simulink subsystem "block_admittance_controller_quat"  (R2021b)
settings: Solver=VariableStepAuto  StartTime=0.0  StopTime=10.0  RelTol=1e-3
undefined symbols (not defined in the file): Kd, Kp, Md, q_d_cd0, w_d_cd0
settings Model: Creator=Martin  LastModifiedBy=Martin

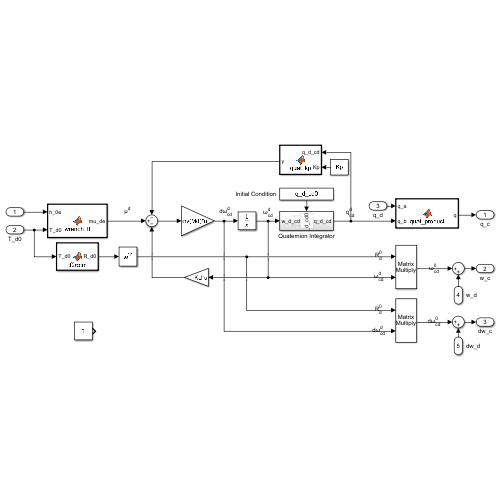
[thumbnail: Simulink's stored preview of the top-level diagram]
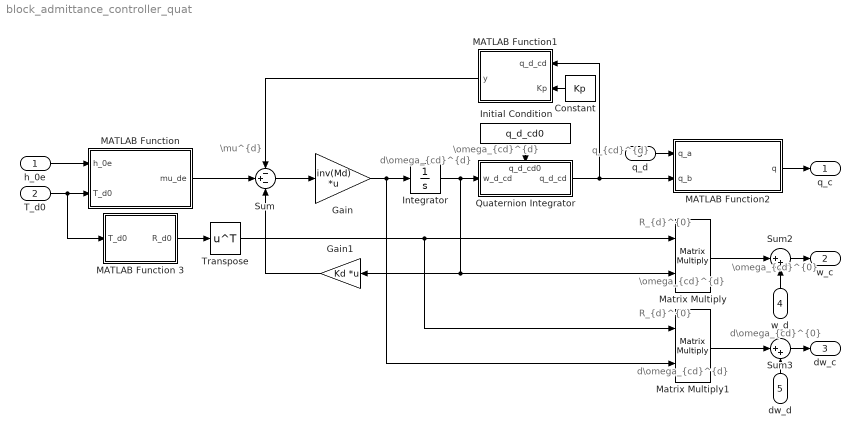
== system block_admittance_controller_quat ==
  note: q_{cd}^{d}
  note: \omega_{cd}^{d}
  note: d\omega_{cd}^{d}
  note: \omega_{cd}^{d}
  note: R_{d}^{0}
  note: \omega_{cd}^{0}
  note: \mu^{d}
  note: R_{d}^{0}
  note: d\omega_{cd}^{d}
  note: d\omega_{cd}^{0}
  h_0e : Inport
  T_d0 : Inport  Port=2
  q_d : Inport  Port=3  PortDimensions=[1 4]
  w_d : Inport  Port=4
  dw_d : Inport  Port=5
  Constant : Constant  Value=Kp  VectorParams1D=off
  Gain : Gain  Gain=inv(Md)  Multiplication=Matrix(K*u)
  Gain1 : Gain  Gain=Kd  Multiplication=Matrix(K*u)
  Initial Condition : Constant  Value=q_d_cd0  VectorParams1D=off
  Integrator : Integrator  InitialCondition=w_d_cd0
  MATLAB Function : MATLAB Function  TreatAsAtomicUnit=on
  MATLAB Function 3 : MATLAB Function  TreatAsAtomicUnit=on
  MATLAB Function1 : MATLAB Function  TreatAsAtomicUnit=on
  MATLAB Function2 : MATLAB Function  TreatAsAtomicUnit=on
  Matrix Multiply : Product  Multiplication=Matrix(*)
  Matrix Multiply1 : Product  Multiplication=Matrix(*)
  Quaternion Integrator : Subsystem
      settings: PortSchema="{\"entries\":[{\"content\":{\"sides\":[{\"content\":{\"connectorIds\":[\"In1\"]},\"type\":\"ConnectorPlacement.EquallySpacedRectSide\",\"uuid\":\"9147276c-c282-42f4-b280-5cb7655f40a2\"},{\"content\":{\"connectorIds\":[\"Out1\"],\"side\":\"RIGHT\"},\"type\":\"ConnectorPlacement.EquallySpacedRectSide\",\"uuid\":\"8158b75f-7283-43f6-a546-44f02f66480d\"},{\"content\":{\"connectorIds\":[\"In2\"],\"side\":\"TOP\"},\"type\":\"ConnectorPlacement.EquallySpacedRectSide\",\"uuid\":\"e337812f-5cf7-40c1-8c1c-b6f28ef83770\"},{\"content\":{\"connectorIds\":[],\"side\":\"BOTTOM\"},\"type\":\"ConnectorPlacement.EquallySpacedRectSide\",\"uuid\":\"6d87eade-312b-4fff-ae27-7548639e2b90\"}]},\"type\":\"ConnectorPlacement.EquallySpacedConnector\",\"uuid\":\"76e88866-094a-46fd-b80c-7282024b89fb\"}],\"packageUris\":[\"http://schema.mathworks.com/mf0/Connector/R2020b\"],\"version\":\"1.0\"}"
  Sum : Sum  Inputs=-+-
  Sum2 : Sum  Inputs=|++
  Sum3 : Sum  Inputs=|++
  Transpose : Math  Operator=transpose  SaturateOnIntegerOverflow=on
  q_c : Outport
  w_c : Outport  Port=2
  dw_c : Outport  Port=3
  wires:
  Sum2/1 -> w_c/1
  Sum3/1 -> dw_c/1
  Gain/1 -> Integrator/1, Matrix Multiply1/2
  w_d/1 -> Sum2/2
  dw_d/1 -> Sum3/2
  Sum/1 -> Gain/1
  Gain1/1 -> Sum/3
  h_0e/1 -> MATLAB Function/1(h_0e)
  MATLAB Function/1(mu_de) -> Sum/2
  T_d0/1 -> MATLAB Function/2(T_d0), MATLAB Function 3/1(T_d0)
  Quaternion Integrator/1(q_d_cd) -> MATLAB Function1/1(q_d_cd), MATLAB Function2/2(q_b)
  Initial Condition/1 -> Quaternion Integrator/2(q_d_cd0)
  MATLAB Function1/1(y) -> Sum/1
  Constant/1 -> MATLAB Function1/2(Kp)
  MATLAB Function2/1(q) -> q_c/1
  q_d/1 -> MATLAB Function2/1(q_a)
  MATLAB Function 3/1(R_d0) -> Transpose/1
  Matrix Multiply/1 -> Sum2/1
  Transpose/1 -> Matrix Multiply/1, Matrix Multiply1/1
  Integrator/1 -> Matrix Multiply/2, Gain1/1, Quaternion Integrator/1(w_d_cd)
  Matrix Multiply1/1 -> Sum3/1

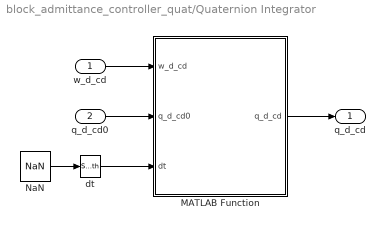
== system block_admittance_controller_quat/Quaternion Integrator ==
  w_d_cd : Inport
  q_d_cd0 : Inport  Port=2
  MATLAB Function : MATLAB Function  TreatAsAtomicUnit=on
  NaN : Constant  Value=NaN  OutDataTypeStr=Inherit: Inherit via back propagation
  dt : SampleTimeMath  TsampMathOp=Ts Only
  q_d_cd : Outport
  wires:
  NaN/1 -> dt/1
  MATLAB Function/1(q_d_cd) -> q_d_cd/1
  w_d_cd/1 -> MATLAB Function/1(w_d_cd)
  dt/1 -> MATLAB Function/3(dt)
  q_d_cd0/1 -> MATLAB Function/2(q_d_cd0)

== matlab function block_admittance_controller_quat/MATLAB Function ==
  data: h_0e input; mu_de output; T_d0 input
function mu_de = wrench_tf(h_0e, T_d0)

    % given end-effector wrench h_0e in base frame
    % transform such that given in desired frame, h_de

    R_d0 = tform2rotm(T_d0);
    t_d0 = tform2trvec(T_d0);
    % Ad   = [R_d0 0 ; skew(t_d0) * R_d0 R_d0];

    mu_de = [skew(t_d0) * R_d0 R_d0] * h_0e; % only for moment

end

== matlab function block_admittance_controller_quat/MATLAB Function1 ==
  data: q_d_cd input; Kp input; y output
function y = quat_kp(q_d_cd, Kp)
    
    % q = [cos(th/2) r * sin(th/2)] = [eta, eps] = [a b c d]
    eta_d_cd = q_d_cd(1); % [a]
    eps_d_cd = q_d_cd(2:4)'; % [b c d]

    E = @(eta, eps) eta * eye(3) - skew(eps);

    Kp_ = 2 * E(eta_d_cd, eps_d_cd)' * Kp;
    y = Kp_ * eps_d_cd;

end

== matlab function block_admittance_controller_quat/MATLAB Function2 ==
  data: q_a input; q output; q_b input
function q = quat_product(q_a, q_b)
    q = compact(quaternion(q_a) * quaternion(q_b));
end

== matlab function block_admittance_controller_quat/MATLAB Function 3 ==
  data: T_d0 input; R_d0 output
function R_d0 = tf2rotm(T_d0)
    R_d0 = T_d0(1:3, 1:3);
end

== matlab function block_admittance_controller_quat/Quaternion Integrator/MATLAB Function ==
  settings: updateMethod=DISCRETE  sampleTime=0.01
  data: w_d_cd input; q_d_cd0 input; q_d_cd output; dt input
function q_d_cd = integrate_quat(w_d_cd, q_d_cd0, dt)
    
    persistent q_d_cd_prev % quaternion()
    if isempty(q_d_cd_prev)
        q_d_cd_prev = quaternion(q_d_cd0);
        q_d_cd = compact(q_d_cd_prev);
        return
    end

    if norm(w_d_cd) == 0 % edge case when input near zero
        q_d_cd = compact(q_d_cd_prev);
        return
    end
    
    qexp = @(r) quaternion([ cos(norm(r)) , [r/norm(r) * sin(norm(r))]' ]);

    q_d_cd_ = qexp(dt/2 * w_d_cd) * q_d_cd_prev;
    q_d_cd_prev = q_d_cd_;

    q_d_cd = compact(q_d_cd_); % output as array

end
